simulink model "SOC_sfun"  (R2024b)
settings: Solver=FixedStepDiscrete  StartTime=0.0  StopTime=inf  RelTol=1e-3  EnableMultiTasking=on
undefined symbols (not defined in the file or in its folder): C_OcvTable, C_SocTable, SOCc_CapacityFilterCoeff, SOCk_CellBalancingResistor, SOCk_CellCapacity, SOCk_HrsToSec, SOCk_NumberInSeries, SOCk_SocMaxPercentage, SOCk_SocMinPercentage, SOCk_stepSize, SOCk_ToFractionFromPercentage, SOCk_ToPercentage, SOCv_factoryInitSohC, SOCv_InitalSOC
settings Model: TunableVars=C_OcvTable,C_SocTable,SOCc_CapacityFilterCoeff,SOCk_CellBalancingResistor,SOCk_CellCapacity,SOCk_HrsToSec,SOCk_NumberInSeries,SOCk_SocMaxPercentage,SOCk_SocMinPercentage,SOCk_ToFractionFromPercentage,SOCk_ToPercentage,SOCk_stepSize,SOCv_InitalSOC,SOCv_factoryInitSohC  TunableVarsStorageClass=Auto,Auto,Auto,Auto,Auto,Auto,Auto,Auto,Auto,Auto,Auto,Auto,Auto,Auto  TunableVarsTypeQualifier=,,,,,,,,,,,,,  Creator=nctzv8  LastModifiedBy=voillat
settings ConfigSet: Description=OpenECU configuration set for code generation under RTW-EC.
settings SolverCC: AlgebraicLoopSolver=TrustRegion  PositivePriorityOrder=on
settings DataIOCC: LimitDataPoints=on  SaveFormat=Array  SignalLoggingSaveFormat=ModelDataLogs
settings OptimizationCC: DefaultParameterBehavior=Inlined  InlineInvariantSignals=on  ExpressionDepthLimit=2147483647  StateBitsets=on  DataBitsets=on  ZeroExternalMemoryAtStartup=off  ZeroInternalMemoryAtStartup=off  NoFixptDivByZeroProtection=on  EfficientFloat2IntCast=on  LifeSpan=1  EfficientTunableParamExpr=on
settings DebuggingCC: SaveWithParameterizedLinksMsg=none  SignalResolutionControl=TryResolveAllWithWarning  MultiTaskDSMMsg=warning  MultiTaskCondExecSysMsg=none  SingleTaskRateTransMsg=error  CheckMatrixSingularityMsg=warning  VectorMatrixConversionMsg=warning  SignalLabelMismatchMsg=warning  UnconnectedInputMsg=warning  UnconnectedOutputMsg=warning  UnconnectedLineMsg=warning  AllowSymbolicDim=off  StateNameClashWarn=warning  SFUnexpectedBacktrackingDiag=warning  SFNoUnconditionalDefaultTransitionDiag=warning  SFExecutionAtInitializationDiag=none  ArithmeticOperatorsInVariantConditions=warning
settings HardwareCC: ProdBitPerPointer=32  ProdBitPerSizeT=32  ProdBitPerPtrDiffT=32  ProdLargestAtomicInteger=Long  ProdLargestAtomicFloat=Double  ProdEndianess=BigEndian  ProdWordSize=32  ProdHWDeviceType=Freescale->32-bit PowerPC  TargetIntDivRoundTo=Zero  TargetEndianess=BigEndian  TargetHWDeviceType=Freescale->32-bit PowerPC  ProdEqTarget=off
settings ModelReferenceCC: EnableRefExpFcnMdlSchedulingChecks=on  PropagateSignalLabelsOutOfModel=off
settings SFSimCC: SimUseLocalCustomCode=off  MATLABDynamicMemAlloc=off  CustomCodeUndefinedFunction=UseInterfaceOnly
settings RTWCC: Description=OpenECU Platform Target (ERT, optimised floating-point code)  SystemTargetFile=openecu_ert.tlc  MakeCommand=make_rtw optimized_floating_point=1  TemplateMakefile=openecu_ert_r2015b_64.tmf  RetainRTWFile=on  RTWUseLocalCustomCode=off  IncludeHyperlinkInReport=on  GPUComputeCapability=3.5
settings CodeAppCC: ForceParamTrailComments=on  IgnoreCustomStorageClasses=off  SimulinkDataObjDesc=on  CustomSymbolStrType=$N$R$M  InsertBlockDesc=on  StateflowObjectComments=on  InternalIdentifier=Classic
settings STFCustomTargetCC: TargetLibSuffix=.a  GenerateSampleERTMain=on  IncludeMdlTerminateFcn=off  CombineOutputUpdateFcns=on  IncludeFileDelimiter=UseQuote  ERTCustomFileBanners=on  SupportContinuousTime=off  RemoveResetFunc=on  MATLABClassNameForMDSCustomization=Simulink.SoftwareTarget.ERTCustomization  SystemTargetFile=openecu_ert.tlc
settings ERTTargetCC: MultiwordLength=2048  GenerateSampleERTMain=on  ParMdlRefBuildCompliant=off  CompOptLevelCompliant=off  ConcurrentExecutionCompliant=off  IncludeMdlTerminateFcn=off  IncludeFileDelimiter=UseQuote  SupportNonInlinedSFcns=on  ModelStepFunctionPrototypeControlCompliant=off  CPPClassGenCompliant=off  UseToolchainInfoCompliant=off  ExtModeMexFile=noextcomm  ERTSrcFileBannerTemplate=oe_code_c_template.cgt  ERTHdrFileBannerTemplate=oe_code_h_template.cgt  ERTDataSrcFileTemplate=oe_data_c_template.cgt  ERTDataHdrFileTemplate=oe_data_h_template.cgt  ERTCustomFileTemplate=example_file_process.tlc  GlobalDataDefinition=InSeparateSourceFile  GlobalDataReference=InSeparateHeaderFile  ConvertIfToSwitch=off  SuppressUnreachableDefaultCases=off  EnableUserReplacementTypes=on  DynamicArrayContainerType=coder::array
settings ConfigComp: CovMetricSettings=dw  CovSaveCumulativeToWorkspaceVar=on  CovSaveSingleToWorkspaceVar=on  CovExternalEMLEnable=off

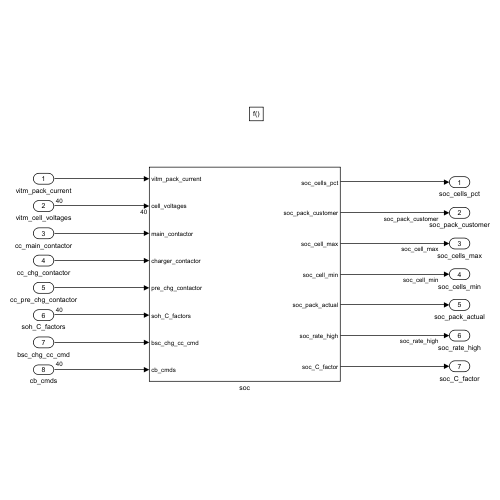
[thumbnail: Simulink's stored preview of the top-level diagram]
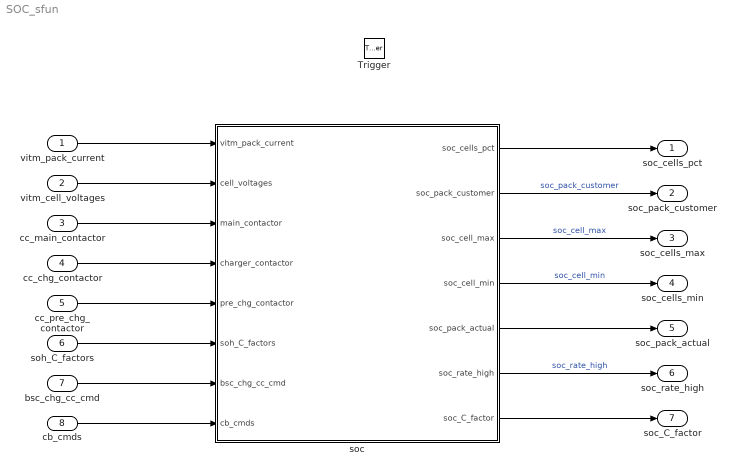
== system SOC_sfun ==
  vitm_pack_current : Inport
  vitm_cell_voltages : Inport  Port=2  PortDimensions=40
  cc_main_contactor : Inport  Port=3
  cc_chg_contactor : Inport  Port=4
  cc_pre_chg_contactor : Inport  Port=5
  soh_C_factors : Inport  Port=6  PortDimensions=40
  bsc_chg_cc_cmd : Inport  Port=7
  cb_cmds : Inport  Port=8  OutDataTypeStr=boolean  PortDimensions=40
  Trigger : TriggerPort  TriggerType=function-call  VariantControl=(inherit)  PortDimensions=1
  soc : Subsystem  mask{prm_to_disp=[1..10], sfcnParam1=C_OcvTable, sfcnParam2=C_SocTable, sfcnParam3=SOCc_CapacityFilterCoeff, sfcnParam4=SOCk_CellBalancingResistor, sfcnParam5=SOCk_CellCapacity, sfcnParam6=SOCk_HrsToSec, sfcnParam7=SOCk_NumberInSeries, sfcnParam8=SOCk_SocMaxPercentage, sfcnParam9=SOCk_SocMinPercentage, sfcnParam10=SOCk_ToFractionFromPercentage, sfcnParam11=SOCk_ToPercentage, sfcnParam12=SOCk_stepSize, sfcnParam13=SOCv_InitalSOC, sfcnParam14=SOCv_factoryInitSohC}
      mask prompts: prm_to_disp "Display S-function Parameters:"; sfcnParam1 "C_OcvTable:"; sfcnParam2 "C_SocTable:"; sfcnParam3 "SOCc_CapacityFilterCoeff:"; sfcnParam4 "SOCk_CellBalancingResistor:"; sfcnParam5 "SOCk_CellCapacity:"; sfcnParam6 "SOCk_HrsToSec:"; sfcnParam7 "SOCk_NumberInSeries:"; sfcnParam8 "SOCk_SocMaxPercentage:"; sfcnParam9 "SOCk_SocMinPercentage:"; sfcnParam10 "SOCk_ToFractionFromPercentage:"; sfcnParam11 "SOCk_ToPercentage:"; sfcnParam12 "SOCk_stepSize:"; sfcnParam13 "SOCv_InitalSOC:"; sfcnParam14 "SOCv_factoryInitSohC:"
      mask help: Simulink:masks:GenSFuncDesc_MD
      mask Help: eval('feval(''rtwprivate'',''rtwhelpview'',''rtw_sfcn_block'')');
      mask TypeOptions prm_to_disp: [1..10] | [11..14]
      mask Callback prm_to_disp: slmaskprmdispcntrl(gcbh)
  soc_cells_pct : Outport
  soc_pack_customer : Outport  Port=2
  soc_cells_max : Outport  Port=3
  soc_cells_min : Outport  Port=4
  soc_pack_actual : Outport  Port=5
  soc_rate_high : Outport  Port=6
  soc_C_factor : Outport  Port=7  InitialOutput=ones(40,1)
  wires:
  vitm_pack_current/1 -> soc/1(vitm_pack_current)
  vitm_cell_voltages/1 -> soc/2(cell_voltages)
  cc_main_contactor/1 -> soc/3(main_contactor)
  cc_pre_chg_contactor/1 -> soc/5(pre_chg_contactor)
  cc_chg_contactor/1 -> soc/4(charger_contactor)
  soh_C_factors/1 -> soc/6(soh_C_factors)
  bsc_chg_cc_cmd/1 -> soc/7(bsc_chg_cc_cmd)
  cb_cmds/1 -> soc/8(cb_cmds)
  soc/1(soc_cells_pct) -> soc_cells_pct/1
  soc/2(soc_pack_customer) -> soc_pack_customer/1  "soc_pack_customer"
  soc/3(soc_cell_max) -> soc_cells_max/1  "soc_cell_max"
  soc/4(soc_cell_min) -> soc_cells_min/1  "soc_cell_min"
  soc/5(soc_pack_actual) -> soc_pack_actual/1
  soc/6(soc_rate_high) -> soc_rate_high/1  "soc_rate_high"
  soc/7(soc_C_factor) -> soc_C_factor/1

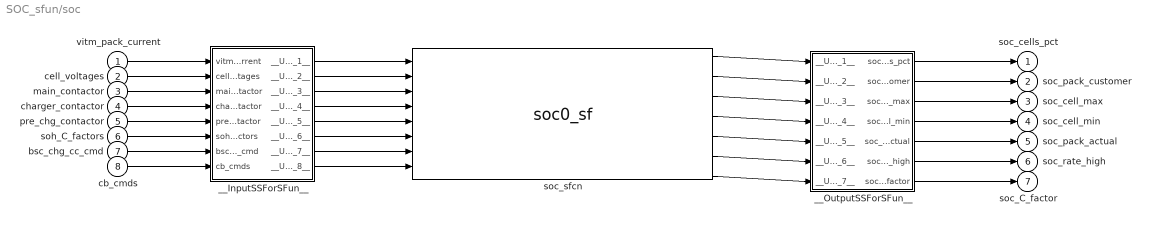
== system SOC_sfun/soc ==
  vitm_pack_current : Inport
  cell_voltages : Inport  Port=2  PortDimensions=40
  main_contactor : Inport  Port=3
  charger_contactor : Inport  Port=4
  pre_chg_contactor : Inport  Port=5
  soh_C_factors : Inport  Port=6
  bsc_chg_cc_cmd : Inport  Port=7
  cb_cmds : Inport  Port=8
  __InputSSForSFun__ : Subsystem
  __OutputSSForSFun__ : Subsystem
  soc_sfcn : S-Function  FunctionName=soc0_sf  Parameters=sfcnParam1, sfcnParam2, sfcnParam3, sfcnParam4, sfcnParam5, sfcnParam6, sfcnParam7, sfcnParam8, sfcnParam9, sfcnParam10, sfcnParam11, sfcnParam12, sfcnParam13, sfcnParam14  SFunctionModules=""  SFunctionDeploymentMode=off  EnableBusSupport=off  mask{rtw_sf_name=soc0_sf, showVar=off, prm_to_disp=[1..10], sfcnParam1=sfcnParam1, sfcnParam2=sfcnParam2, sfcnParam3=sfcnParam3, sfcnParam4=sfcnParam4, sfcnParam5=sfcnParam5, sfcnParam6=sfcnParam6, sfcnParam7=sfcnParam7, sfcnParam8=sfcnParam8, sfcnParam9=sfcnParam9, sfcnParam10=sfcnParam10, sfcnParam11=sfcnParam11, sfcnParam12=sfcnParam12, sfcnParam13=sfcnParam13, sfcnParam14=sfcnParam14}
      mask prompts: rtw_sf_name "Simulink:masks:GenSFuncName_MP"; showVar "Simulink:masks:GenSFuncShowModuleList_MP"; prm_to_disp "Display S-function Parameters:"; sfcnParam1 "C_OcvTable:"; sfcnParam2 "C_SocTable:"; sfcnParam3 "SOCc_CapacityFilterCoeff:"; sfcnParam4 "SOCk_CellBalancingResistor:"; sfcnParam5 "SOCk_CellCapacity:"; sfcnParam6 "SOCk_HrsToSec:"; sfcnParam7 "SOCk_NumberInSeries:"; sfcnParam8 "SOCk_SocMaxPercentage:"; sfcnParam9 "SOCk_SocMinPercentage:"; sfcnParam10 "SOCk_ToFractionFromPercentage:"; sfcnParam11 "SOCk_ToPercentage:"; sfcnParam12 "SOCk_stepSize:"; sfcnParam13 "SOCv_InitalSOC:"; sfcnParam14 "SOCv_factoryInitSohC:"
      mask help: Simulink:masks:GenSFuncDesc_MD
      mask init:
      | displist = '';
      | if ~strcmp(get_param(gcb, 'FunctionName'), rtw_sf_name);
      |   set_param(gcb, 'FunctionName', rtw_sf_name);
      | end
      | % Check if we are generating code
      | rtw_mode = false;
      | if strcmpi(get_param(bdroot(gcb),'SimulationStatus'),'Initializing')
      | 	rtw_mode = strcmpi(get_param(bdroot(gcb),'BuildingRTWCode'),'on') && ...
      | 		~strcmpi(get_param(bdroot(gcb),'TargetStyle'),'SimulationTarget');
      | end
      | if showVar || rtw_mode
      | 	if exist('rtwsfunc') == 2 | exist('rtwsfunc') == 6
      | 		tmplist = rtwsfunc(rtw_sf_name,gcb);
      | 		tmplist = DAStudio.message('Simulink:masks:GenSFuncListOfModules_IC', tmplist);
      | 	elseif showVar
      | 		tmplist1 = DAStudio.message('Simulink:masks:GenSFuncListOfModules_IC', '');
      |         tmplist2 = DAStudio.message('Simulink:masks:GenSFuncNotLicensed_IC');
      |         tmplist = [tmplist1 tmplist2];
      |  	end
      | end
      | if showVar
      |   displist = tmplist;
      | end
      settings: CopyFcn=|
      | if ~strcmp(get_param(gcb,'Linkstatus'),'none') && ...
      | ~strcmp(get_param(gcb,'Linkstatus'),'implicit')
      |   set_param(gcb,'LinkStatus','none');
      | end
      mask Help: eval('feval(''rtwprivate'',''rtwhelpview'',''rtw_sfcn_block'')');
      mask TypeOptions prm_to_disp: [1..10] | [11..14]
      mask Callback prm_to_disp: slmaskprmdispcntrl(gcbh)
      mask Display:
      | port_label('input',1,'vitm_pack_current');
      | port_label('input',2,'cell_voltages');
      | port_label('input',3,'main_contactor');
      | port_label('input',4,'charger_contactor');
      | port_label('input',5,'pre_chg_contactor');
      | port_label('input',6,'soh_C_factors');
      | port_label('input',7,'bsc_chg_cc_cmd');
      | port_label('input',8,'cb_cmds');
      | port_label('output',1,'soc_cells_pct');
      | port_label('output',2,'soc_pack_customer');
      | port_label('output',3,'soc_cell_max');
      | port_label('output',4,'soc_cell_min');
      | port_label('output',5,'soc_pack_actual');
      | port_label('output',6,'soc_rate_high');
      | port_label('output',7,'soc_C_factor');
  soc_cells_pct : Outport
  soc_pack_customer : Outport  Port=2
  soc_cell_max : Outport  Port=3
  soc_cell_min : Outport  Port=4
  soc_pack_actual : Outport  Port=5
  soc_rate_high : Outport  Port=6
  soc_C_factor : Outport  Port=7
  wires:
  vitm_pack_current/1 -> __InputSSForSFun__/1(vitm_pack_current)
  cell_voltages/1 -> __InputSSForSFun__/2(cell_voltages)
  main_contactor/1 -> __InputSSForSFun__/3(main_contactor)
  charger_contactor/1 -> __InputSSForSFun__/4(charger_contactor)
  pre_chg_contactor/1 -> __InputSSForSFun__/5(pre_chg_contactor)
  soh_C_factors/1 -> __InputSSForSFun__/6(soh_C_factors)
  bsc_chg_cc_cmd/1 -> __InputSSForSFun__/7(bsc_chg_cc_cmd)
  cb_cmds/1 -> __InputSSForSFun__/8(cb_cmds)
  __InputSSForSFun__/1(__UniqueOutportName__1__) -> soc_sfcn/1
  __InputSSForSFun__/2(__UniqueOutportName__2__) -> soc_sfcn/2
  __InputSSForSFun__/3(__UniqueOutportName__3__) -> soc_sfcn/3
  __InputSSForSFun__/4(__UniqueOutportName__4__) -> soc_sfcn/4
  __InputSSForSFun__/5(__UniqueOutportName__5__) -> soc_sfcn/5
  __InputSSForSFun__/6(__UniqueOutportName__6__) -> soc_sfcn/6
  __InputSSForSFun__/7(__UniqueOutportName__7__) -> soc_sfcn/7
  __InputSSForSFun__/8(__UniqueOutportName__8__) -> soc_sfcn/8
  soc_sfcn/1 -> __OutputSSForSFun__/1(__UniqueInportName__1__)
  soc_sfcn/2 -> __OutputSSForSFun__/2(__UniqueInportName__2__)
  soc_sfcn/3 -> __OutputSSForSFun__/3(__UniqueInportName__3__)
  soc_sfcn/4 -> __OutputSSForSFun__/4(__UniqueInportName__4__)
  soc_sfcn/5 -> __OutputSSForSFun__/5(__UniqueInportName__5__)
  soc_sfcn/6 -> __OutputSSForSFun__/6(__UniqueInportName__6__)
  soc_sfcn/7 -> __OutputSSForSFun__/7(__UniqueInportName__7__)
  __OutputSSForSFun__/1(soc_cells_pct) -> soc_cells_pct/1
  __OutputSSForSFun__/2(soc_pack_customer) -> soc_pack_customer/1
  __OutputSSForSFun__/3(soc_cell_max) -> soc_cell_max/1
  __OutputSSForSFun__/4(soc_cell_min) -> soc_cell_min/1
  __OutputSSForSFun__/5(soc_pack_actual) -> soc_pack_actual/1
  __OutputSSForSFun__/6(soc_rate_high) -> soc_rate_high/1
  __OutputSSForSFun__/7(soc_C_factor) -> soc_C_factor/1

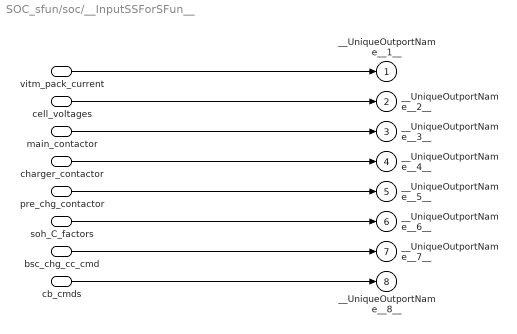
== system SOC_sfun/soc/__InputSSForSFun__ ==
  vitm_pack_current : Inport
  cell_voltages : Inport  Port=2  PortDimensions=40
  main_contactor : Inport  Port=3
  charger_contactor : Inport  Port=4
  pre_chg_contactor : Inport  Port=5
  soh_C_factors : Inport  Port=6
  bsc_chg_cc_cmd : Inport  Port=7
  cb_cmds : Inport  Port=8
  __UniqueOutportName__1__ : Outport
  __UniqueOutportName__2__ : Outport  Port=2
  __UniqueOutportName__3__ : Outport  Port=3
  __UniqueOutportName__4__ : Outport  Port=4
  __UniqueOutportName__5__ : Outport  Port=5
  __UniqueOutportName__6__ : Outport  Port=6
  __UniqueOutportName__7__ : Outport  Port=7
  __UniqueOutportName__8__ : Outport  Port=8
  wires:
  vitm_pack_current/1 -> __UniqueOutportName__1__/1
  cell_voltages/1 -> __UniqueOutportName__2__/1
  main_contactor/1 -> __UniqueOutportName__3__/1
  charger_contactor/1 -> __UniqueOutportName__4__/1
  pre_chg_contactor/1 -> __UniqueOutportName__5__/1
  soh_C_factors/1 -> __UniqueOutportName__6__/1
  bsc_chg_cc_cmd/1 -> __UniqueOutportName__7__/1
  cb_cmds/1 -> __UniqueOutportName__8__/1

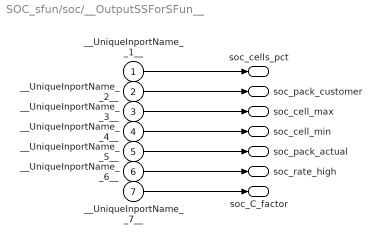
== system SOC_sfun/soc/__OutputSSForSFun__ ==
  __UniqueInportName__1__ : Inport
  __UniqueInportName__2__ : Inport  Port=2
  __UniqueInportName__3__ : Inport  Port=3
  __UniqueInportName__4__ : Inport  Port=4
  __UniqueInportName__5__ : Inport  Port=5
  __UniqueInportName__6__ : Inport  Port=6
  __UniqueInportName__7__ : Inport  Port=7
  soc_cells_pct : Outport
  soc_pack_customer : Outport  Port=2
  soc_cell_max : Outport  Port=3
  soc_cell_min : Outport  Port=4
  soc_pack_actual : Outport  Port=5
  soc_rate_high : Outport  Port=6
  soc_C_factor : Outport  Port=7
  wires:
  __UniqueInportName__1__/1 -> soc_cells_pct/1
  __UniqueInportName__2__/1 -> soc_pack_customer/1
  __UniqueInportName__3__/1 -> soc_cell_max/1
  __UniqueInportName__4__/1 -> soc_cell_min/1
  __UniqueInportName__5__/1 -> soc_pack_actual/1
  __UniqueInportName__6__/1 -> soc_rate_high/1
  __UniqueInportName__7__/1 -> soc_C_factor/1
